simulink model "zad91simulink"  (R2023a)
settings: Solver=VariableStepAuto  StartTime=0.0  StopTime=10.0  RelTol=1e-3
values from neighbouring files (symbols this model uses):
  L_np_rz = acker(A_22', A_12', [b_obsv_np_rz, b_obsv_np_rz])'    [zad91.m]
  u_multiply = B_2 - L_np_rz*B_1    [zad91.m]
  w_multiply = (A_22 - L_np_rz*A_12)    [zad91.m]
  y_multiply = A_21 - L_np_rz*A_11    [zad91.m]
settings Model: Creator=pkutyl  LastModifiedBy=pkutyl

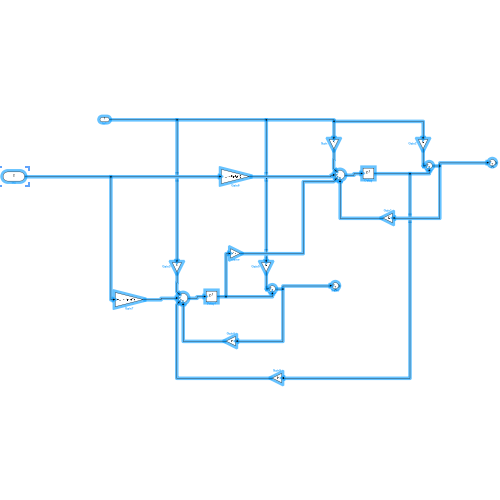
[thumbnail: Simulink's stored preview of the top-level diagram]
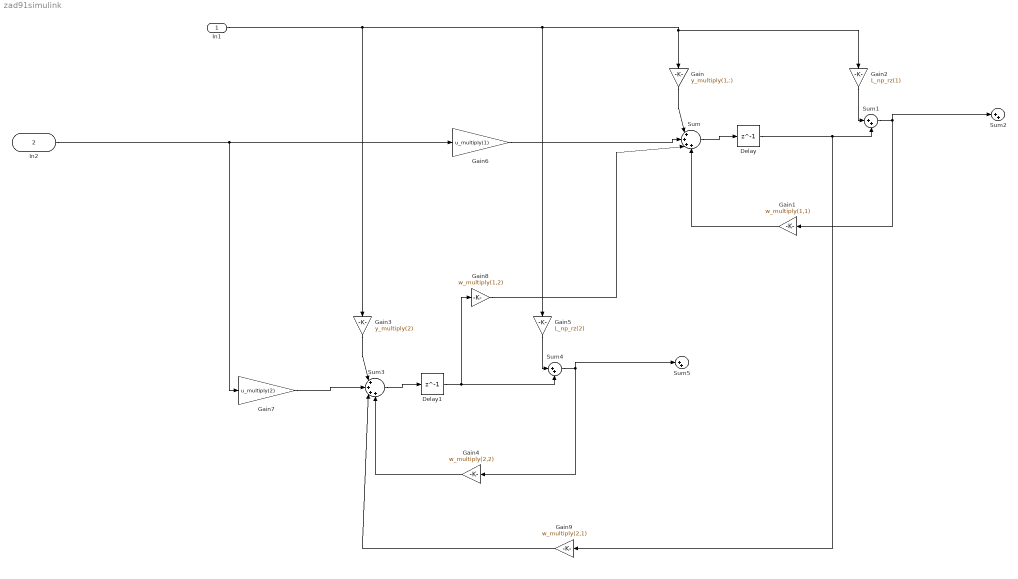
== system zad91simulink ==
  In1 : Inport
  In2 : Inport  Port=2
  Delay : Delay  DelayLength=1  InitialCondition=0
  Delay1 : Delay  DelayLength=1  InitialCondition=0
  Gain : Gain  Gain=y_multiply(1,:)
  Gain1 : Gain  Gain=w_multiply(1,1)
  Gain2 : Gain  Gain=L_np_rz(1)
  Gain3 : Gain  Gain=y_multiply(2)
  Gain4 : Gain  Gain=w_multiply(2,2)
  Gain5 : Gain  Gain=L_np_rz(2)
  Gain6 : Gain  Gain=u_multiply(1)
  Gain7 : Gain  Gain=u_multiply(2)
  Gain8 : Gain  Gain=w_multiply(1,2)
  Gain9 : Gain  Gain=w_multiply(2,1)
  Sum : Sum  Inputs=|++++
  Sum{1..2,4..5} (4 alike) : Sum  Inputs=|++
  Sum3 : Sum  Inputs=|++++
  wires:
  Sum/1 -> Delay/1
  Gain/1 -> Sum/1
  Gain2/1 -> Sum1/1
  Delay/1 -> Gain9/1, Sum1/2
  In1/1 -> Gain5/1, Gain/1, Gain2/1, Gain3/1
  Sum1/1 -> Sum2/1, Gain1/1
  In2/1 -> Gain7/1, Gain6/1
  Gain6/1 -> Sum/2
  Gain1/1 -> Sum/4
  Sum3/1 -> Delay1/1
  Gain3/1 -> Sum3/1
  Sum4/1 -> Sum5/1, Gain4/1
  Gain5/1 -> Sum4/1
  Gain4/1 -> Sum3/4
  Gain7/1 -> Sum3/2
  Delay1/1 -> Gain8/1, Sum4/2
  Gain8/1 -> Sum/3
  Gain9/1 -> Sum3/3
